simulink model "cartPendulumR2018a"  (R2018a)
settings: Solver=ode45  StartTime=0.0  StopTime=P.t_end  RelTol=1e-3  EnableMultiTasking=on
undefined symbols (not defined in the file or in its folder): cartPendulumAnimation, P
settings Model: Creator=beard  LastModifiedBy=rushik
settings DataIOCC: LimitDataPoints=on  SaveFormat=Array  SignalLoggingSaveFormat=ModelDataLogs
settings OptimizationCC: ExpressionDepthLimit=2147483647  InitFltsAndDblsToZero=on  LifeSpan=inf
settings DebuggingCC: UnderspecifiedInitializationDetection=Classic  MergeDetectMultiDrivingBlocksExec=none  SolverPrmCheckMsg=warning  FcnCallInpInsideContextMsg=warning  StateNameClashWarn=warning  SFUnexpectedBacktrackingDiag=warning  SFNoUnconditionalDefaultTransitionDiag=warning  SFExecutionAtInitializationDiag=none
settings HardwareCC: ProdBitPerPointer=32  ProdBitPerSizeT=32  ProdBitPerPtrDiffT=32  ProdLargestAtomicFloat=None  ProdIntDivRoundTo=Undefined  ProdEndianess=Unspecified  ProdWordSize=32  ProdHWDeviceType=32-bit Generic
settings ModelReferenceCC: PropagateSignalLabelsOutOfModel=off
settings CodeAppCC: StateflowObjectComments=on
settings GRTTargetCC: TargetLangStandard=C89/C90 (ANSI)  CombineOutputUpdateFcns=off  GRTInterface=on
settings ConfigComp: CovMetricSettings=dw  CovHtmlReporting=on  CovSaveCumulativeToWorkspaceVar=on  CovSaveSingleToWorkspaceVar=on  CovExternalEMLEnable=off

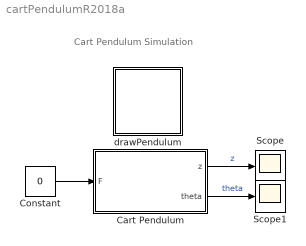
== system cartPendulumR2018a ==
  note: Cart Pendulum Simulation
  Cart Pendulum : Subsystem
  Constant : Constant  Value=0
  Scope : Scope
  Scope1 : Scope
  drawPendulum : Subsystem
      mask Display: image(imread('cartPendulumImage.PNG'))
  wires:
  Cart Pendulum/1(z) -> Scope/1  "z"
  Cart Pendulum/2(theta) -> Scope1/1  "theta"
  Constant/1 -> Cart Pendulum/1(F)

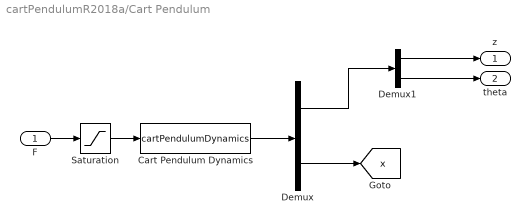
== system cartPendulumR2018a/Cart Pendulum ==
  F : Inport
  Cart Pendulum Dynamics : S-Function  FunctionName=cartPendulumDynamics  Parameters=P  SFunctionDeploymentMode=off  EnableBusSupport=off
  Demux : Demux  Outputs=[2;4]
  Demux1 : Demux  Outputs=2
  Saturation : Saturate  UpperLimit=P.F_max  LowerLimit=-P.F_max
  z : Outport  VectorParamsAs1DForOutWhenUnconnected=off
  theta : Outport  Port=2  VectorParamsAs1DForOutWhenUnconnected=off
  tag scope: x=global
  wires:
  F/1 -> Saturation/1
  Cart Pendulum Dynamics/1 -> Demux/1
  Demux/2 -> [x]
  Demux/1 -> Demux1/1
  Demux1/1 -> z/1
  Demux1/2 -> theta/1
  Saturation/1 -> Cart Pendulum Dynamics/1

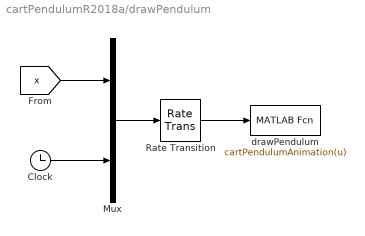
== system cartPendulumR2018a/drawPendulum ==
  Clock : Clock
  Mux : Mux  Inputs=2
  Rate Transition : RateTransition  OutPortSampleTime=P.t_plot
  drawPendulum : MATLABFcn  MATLABFcn=cartPendulumAnimation(u)  OutputDimensions=0
  wires:
  Mux/1 -> Rate Transition/1
  [x] -> Mux/1
  Clock/1 -> Mux/2
  Rate Transition/1 -> drawPendulum/1
